simulink model "COHERENT_MODEM_WITH_LOGIC"  (R2021b)
settings: Solver=VariableStepAuto  StartTime=0.0  StopTime=0.04*5  RelTol=1e-3
values from neighbouring files (symbols this model uses):
  fcarrier = 20000    [run_modem.m]
libraries: dspswit3 x5, dsparch4 x2, simulink x1
settings Model: Creator=hp  LastModifiedBy=caccolillo
settings SolverCC: AlgebraicLoopSolver=TrustRegion
settings DataIOCC: ReturnWorkspaceOutputs=off
settings DebuggingCC: SFMachineParentedDataDiag=warning  ArithmeticOperatorsInVariantConditions=warning
settings SFSimCC: SimUseLocalCustomCode=off  CustomCodeUndefinedFunction=UseInterfaceOnly
settings RTWCC: RTWUseLocalCustomCode=off

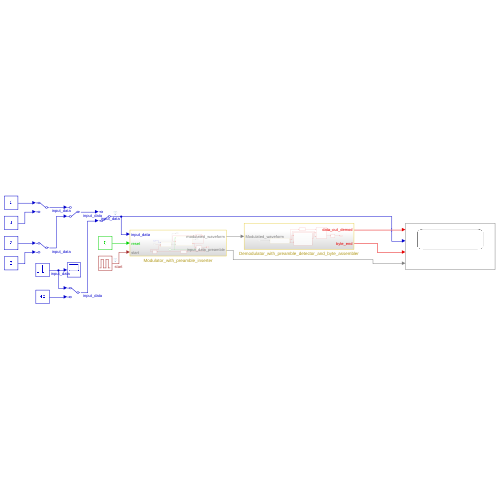
[thumbnail: Simulink's stored preview of the top-level diagram]
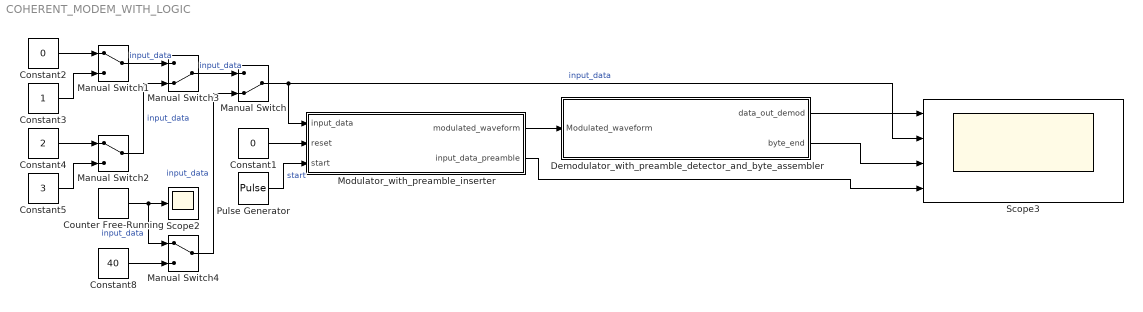
== system COHERENT_MODEM_WITH_LOGIC ==
  Constant1 : Constant  Value=0  OutDataTypeStr=double  SampleTime=1/20000
  Constant2 : Constant  Value=0  OutDataTypeStr=fixdt(0,2)  SampleTime=4/fcarrier
  Constant3 : Constant  OutDataTypeStr=fixdt(0,2)  SampleTime=4/fcarrier
  Constant4 : Constant  Value=2  OutDataTypeStr=fixdt(0,2)  SampleTime=4/fcarrier
  Constant5 : Constant  Value=3  OutDataTypeStr=fixdt(0,2)  SampleTime=4/fcarrier
  Constant8 : Constant  Value=40  OutDataTypeStr=fixdt(0,8)  SampleTime=4/fcarrier
  Counter Free-Running : simulink/Sources/Counter Free-Running  NumBits=8  tsamp=4/fcarrier
  Demodulator_with_preamble_detector_and_byte_assembler : Subsystem
  Manual Switch : ManualSwitch  CurrentSetting=0
  Manual Switch1 : ManualSwitch
  Manual Switch2 : ManualSwitch
  Manual Switch3 : ManualSwitch  CurrentSetting=0
  Manual Switch4 : ManualSwitch
  Modulator_with_preamble_inserter : Subsystem
  Pulse Generator : DiscretePulseGenerator  PulseType=Time based  Period=180/fcarrier  PulseWidth=5
  Scope2 : Scope
  Scope3 : Scope  NumInputPorts=4
  wires:
  Counter Free-Running/1 -> Scope2/1, Manual Switch4/1  "input_data"
  Pulse Generator/1 -> Modulator_with_preamble_inserter/3(start)  "start"
  Modulator_with_preamble_inserter/2(input_data_preamble) -> Scope3/4
  Demodulator_with_preamble_detector_and_byte_assembler/2(byte_end) -> Scope3/3
  Constant1/1 -> Modulator_with_preamble_inserter/2(reset)
  Modulator_with_preamble_inserter/1(modulated_waveform) -> Demodulator_with_preamble_detector_and_byte_assembler/1(Modulated_waveform)
  Manual Switch/1 -> Modulator_with_preamble_inserter/1(input_data), Scope3/2  "input_data"
  Manual Switch4/1 -> Manual Switch/2  "input_data"
  Constant4/1 -> Manual Switch2/1
  Demodulator_with_preamble_detector_and_byte_assembler/1(data_out_demod) -> Scope3/1
  Constant2/1 -> Manual Switch1/1
  Constant8/1 -> Manual Switch4/2
  Constant5/1 -> Manual Switch2/2
  Constant3/1 -> Manual Switch1/2
  Manual Switch3/1 -> Manual Switch/1  "input_data"
  Manual Switch2/1 -> Manual Switch3/2  "input_data"
  Manual Switch1/1 -> Manual Switch3/1  "input_data"

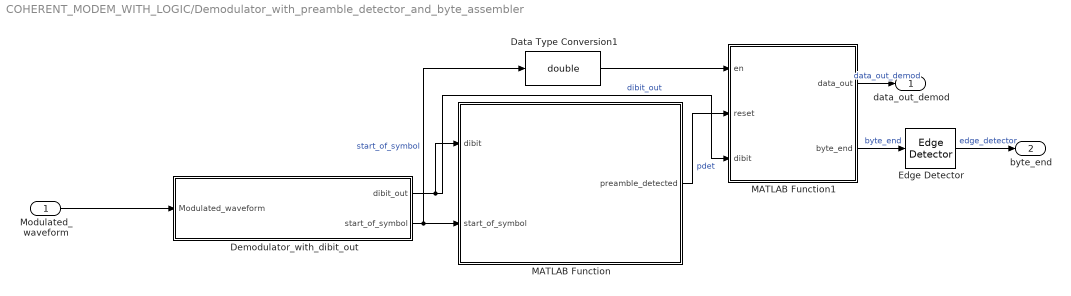
== system COHERENT_MODEM_WITH_LOGIC/Demodulator_with_preamble_detector_and_byte_assembler ==
  Modulated_waveform : Inport
  Data Type Conversion1 : DataTypeConversion  OutDataTypeStr=double
  Demodulator_with_dibit_out : Subsystem
  Edge Detector : dspswit3/Edge Detector  InputProcessing=Columns as channels (frame based)
      settings: SourceProductBaseCode=DS
  MATLAB Function : MATLAB Function  TreatAsAtomicUnit=on
  MATLAB Function1 : MATLAB Function  TreatAsAtomicUnit=on
  data_out_demod : Outport
  byte_end : Outport  Port=2
  wires:
  Demodulator_with_dibit_out/1(dibit_out) -> MATLAB Function/1(dibit), MATLAB Function1/3(dibit)  "dibit_out"
  Demodulator_with_dibit_out/2(start_of_symbol) -> MATLAB Function/2(start_of_symbol), Data Type Conversion1/1  "start_of_symbol"
  Edge Detector/1 -> byte_end/1  "edge_detector"
  Modulated_waveform/1 -> Demodulator_with_dibit_out/1(Modulated_waveform)
  MATLAB Function/1(preamble_detected) -> MATLAB Function1/2(reset)  "pdet"
  Data Type Conversion1/1 -> MATLAB Function1/1(en)
  MATLAB Function1/1(data_out) -> data_out_demod/1  "data_out_demod"
  MATLAB Function1/2(byte_end) -> Edge Detector/1  "byte_end"

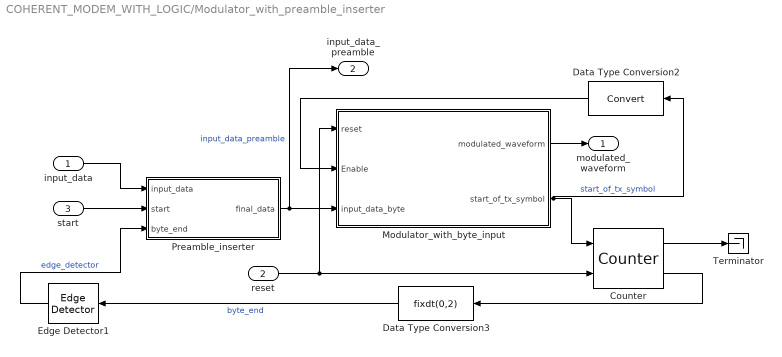
== system COHERENT_MODEM_WITH_LOGIC/Modulator_with_preamble_inserter ==
  input_data : Inport
  reset : Inport  Port=2
  start : Inport  Port=3
  Counter : dspswit3/Counter  Direction=Up  CountEvent=Rising edge  CounterSize=User defined  MaxCount=7  InitialCount=0  Output=Count and Hit  HitValue=7  ResetInput=on  SamplesPerFrame=1  Ts=1  CntDtype=double  HitDtype=Logical
  Data Type Conversion2 : DataTypeConversion
  Data Type Conversion3 : DataTypeConversion  OutMin=[0]  OutMax=[1]  OutDataTypeStr=fixdt(0,2)
  Edge Detector1 : dspswit3/Edge Detector  InputProcessing=Columns as channels (frame based)
      settings: SourceProductBaseCode=DS
  Modulator_with_byte_input : Subsystem
  Preamble_inserter : Subsystem
  Terminator : Terminator
  modulated_waveform : Outport
  input_data_preamble : Outport  Port=2
  wires:
  Preamble_inserter/1(final_data) -> Modulator_with_byte_input/3(input_data_byte), input_data_preamble/1  "input_data_preamble"
  reset/1 -> Counter/2, Modulator_with_byte_input/1(reset)
  Counter/2 -> Data Type Conversion3/1
  Counter/1 -> Terminator/1
  Edge Detector1/1 -> Preamble_inserter/3(byte_end)  "edge_detector"
  start/1 -> Preamble_inserter/2(start)
  Modulator_with_byte_input/2(start_of_tx_symbol) -> Counter/1, Data Type Conversion2/1  "start_of_tx_symbol"
  input_data/1 -> Preamble_inserter/1(input_data)
  Data Type Conversion3/1 -> Edge Detector1/1  "byte_end"
  Data Type Conversion2/1 -> Modulator_with_byte_input/2(Enable)
  Modulator_with_byte_input/1(modulated_waveform) -> modulated_waveform/1

== system COHERENT_MODEM_WITH_LOGIC/Demodulator_with_preamble_detector_and_byte_assembler/Demodulator_with_dibit_out ==
  Modulated_waveform : Inport
  Convert_to_decimal : Subsystem
  Demodulator_with_output_register : Subsystem
  dibit_out : Outport
  start_of_symbol : Outport  Port=2
  wires:
  Demodulator_with_output_register/1(i_demod) -> Convert_to_decimal/2(bit1)
  Demodulator_with_output_register/2(q_demod) -> Convert_to_decimal/1(bit0)
  Convert_to_decimal/1(convert) -> dibit_out/1  "dibit_out"
  Demodulator_with_output_register/3(start_of_symbol) -> start_of_symbol/1
  Modulated_waveform/1 -> Demodulator_with_output_register/1(Modulated_waveform)

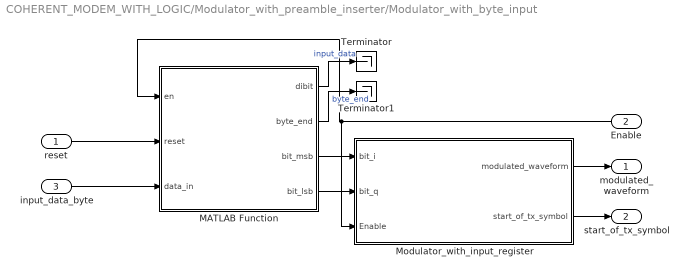
== system COHERENT_MODEM_WITH_LOGIC/Modulator_with_preamble_inserter/Modulator_with_byte_input ==
  reset : Inport
  Enable : Inport  Port=2
  input_data_byte : Inport  Port=3
  MATLAB Function : MATLAB Function  TreatAsAtomicUnit=on
  Modulator_with_input_register : Subsystem
  Terminator : Terminator
  Terminator1 : Terminator
  modulated_waveform : Outport
  start_of_tx_symbol : Outport  Port=2
  wires:
  Enable/1 -> MATLAB Function/1(en), Modulator_with_input_register/3(Enable)
  MATLAB Function/2(byte_end) -> Terminator1/1  "byte_end"
  Modulator_with_input_register/2(start_of_tx_symbol) -> start_of_tx_symbol/1
  input_data_byte/1 -> MATLAB Function/3(data_in)
  reset/1 -> MATLAB Function/2(reset)
  MATLAB Function/1(dibit) -> Terminator/1  "input_data"
  MATLAB Function/4(bit_lsb) -> Modulator_with_input_register/2(bit_q)
  Modulator_with_input_register/1(modulated_waveform) -> modulated_waveform/1
  MATLAB Function/3(bit_msb) -> Modulator_with_input_register/1(bit_i)

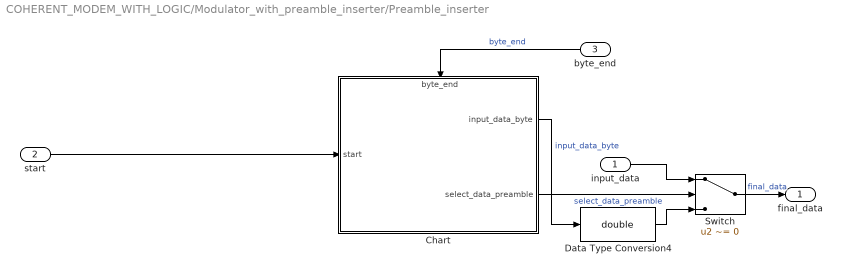
== system COHERENT_MODEM_WITH_LOGIC/Modulator_with_preamble_inserter/Preamble_inserter ==
  input_data : Inport
  start : Inport  Port=2
  byte_end : Inport  Port=3
  Chart : Stateflow chart  TreatAsAtomicUnit=on
      settings: PortSchema="{\"entries\":[{\"content\":{\"sides\":[{\"content\":{\"connectorIds\":[\"In2\"]},\"type\":\"ConnectorPlacement.EquallySpacedRectSide\",\"uuid\":\"c7ea0b9c-d106-4bd1-82e3-4c4e9722273c\"},{\"content\":{\"connectorIds\":[\"Out1\",\"Out2\"],\"side\":\"RIGHT\"},\"type\":\"ConnectorPlacement.EquallySpacedRectSide\",\"uuid\":\"4cc951b6-537b-4e23-ae77-107cf1cb9d20\"},{\"content\":{\"connectorIds\":[\"In1\"],\"side\":\"TOP\"},\"type\":\"ConnectorPlacement.EquallySpacedRectSide\",\"uuid\":\"96187a88-f84a-4d19-a7a7-49870645ca9d\"}]},\"type\":\"ConnectorPlacement.EquallySpacedConnector\",\"uuid\":\"a478a027-a6f7-4a96-ae1b-a22c0dc62afa\"}],\"packageUris\":[\"http://schema.mathworks.com/mf0/Connector/R2020b\"],\"version\":\"1.0\"}"
  Data Type Conversion4 : DataTypeConversion  OutMin=[0]  OutMax=[1]  OutDataTypeStr=double
  Switch : Switch  Criteria=u2 ~= 0  Threshold=1
  final_data : Outport
  wires:
  Switch/1 -> final_data/1  "final_data"
  input_data/1 -> Switch/1
  Data Type Conversion4/1 -> Switch/3
  Chart/2(select_data_preamble) -> Switch/2  "select_data_preamble"
  byte_end/1 -> Chart/1(byte_end)  "byte_end"
  Chart/1(input_data_byte) -> Data Type Conversion4/1  "input_data_byte"
  start/1 -> Chart/2(start)

== system COHERENT_MODEM_WITH_LOGIC/Demodulator_with_preamble_detector_and_byte_assembler/Demodulator_with_dibit_out/Convert_to_decimal ==
  bit0 : Inport
  bit1 : Inport  Port=2
  Add : Sum
  Gain1 : Gain  Gain=2
  convert : Outport
  wires:
  bit1/1 -> Gain1/1
  bit0/1 -> Add/1
  Add/1 -> convert/1  "convert"
  Gain1/1 -> Add/2

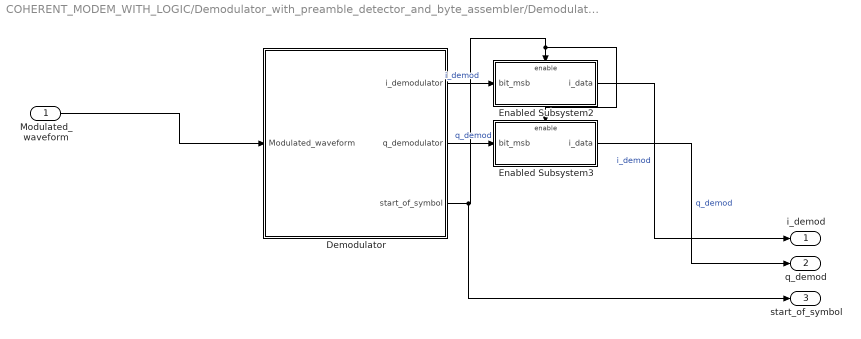
== system COHERENT_MODEM_WITH_LOGIC/Demodulator_with_preamble_detector_and_byte_assembler/Demodulator_with_dibit_out/Demodulator_with_output_register ==
  Modulated_waveform : Inport
  Demodulator : Subsystem
  Enabled Subsystem2 : Subsystem  TreatAsAtomicUnit=on
  Enabled Subsystem3 : Subsystem  TreatAsAtomicUnit=on
  i_demod : Outport
  q_demod : Outport  Port=2
  start_of_symbol : Outport  Port=3
  wires:
  Demodulator/2(q_demodulator) -> Enabled Subsystem3/1(bit_msb)  "q_demod"
  Demodulator/3(start_of_symbol) -> start_of_symbol/1, Enabled Subsystem3/Enable, Enabled Subsystem2/Enable
  Modulated_waveform/1 -> Demodulator/1(Modulated_waveform)
  Demodulator/1(i_demodulator) -> Enabled Subsystem2/1(bit_msb)  "i_demod"
  Enabled Subsystem2/1(i_data) -> i_demod/1  "i_demod"
  Enabled Subsystem3/1(i_data) -> q_demod/1  "q_demod"

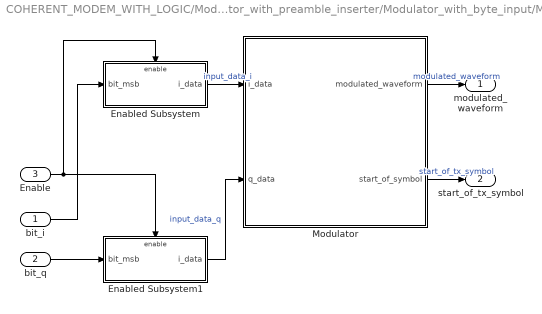
== system COHERENT_MODEM_WITH_LOGIC/Modulator_with_preamble_inserter/Modulator_with_byte_input/Modulator_with_input_register ==
  bit_i : Inport
  bit_q : Inport  Port=2
  Enable : Inport  Port=3
  Enabled Subsystem : Subsystem  TreatAsAtomicUnit=on
  Enabled Subsystem1 : Subsystem  TreatAsAtomicUnit=on
  Modulator : Subsystem
  modulated_waveform : Outport
  start_of_tx_symbol : Outport  Port=2
  wires:
  Enabled Subsystem/1(i_data) -> Modulator/1(i_data)  "input_data_i"
  Modulator/2(start_of_symbol) -> start_of_tx_symbol/1  "start_of_tx_symbol"
  bit_q/1 -> Enabled Subsystem1/1(bit_msb)
  bit_i/1 -> Enabled Subsystem/1(bit_msb)
  Enabled Subsystem1/1(i_data) -> Modulator/2(q_data)  "input_data_q"
  Modulator/1(modulated_waveform) -> modulated_waveform/1  "modulated_waveform"
  Enable/1 -> Enabled Subsystem/Enable, Enabled Subsystem1/Enable

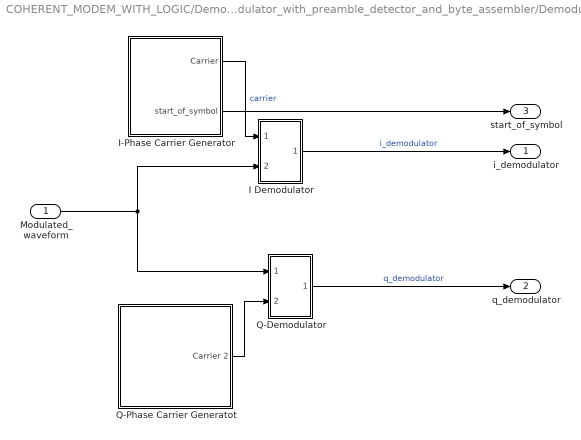
== system COHERENT_MODEM_WITH_LOGIC/Demodulator_with_preamble_detector_and_byte_assembler/Demodulator_with_dibit_out/Demodulator_with_output_register/Demodulator ==
  Modulated_waveform : Inport
  "I Demodulator " : Subsystem
  "I-Phase Carrier Generator " : Subsystem
  Q-Demodulator : Subsystem
  Q-Phase Carrier Generatot : Subsystem
  i_demodulator : Outport
  q_demodulator : Outport  Port=2
  start_of_symbol : Outport  Port=3
  wires:
  Q-Demodulator/1(Out1) -> q_demodulator/1  "q_demodulator"
  Modulated_waveform/1 -> Q-Demodulator/1(In1), "I Demodulator "/2(In2)
  Q-Phase Carrier Generatot/1("Carrier 2 ") -> Q-Demodulator/2("Carrier 2 ")
  "I Demodulator "/1(Out1) -> i_demodulator/1  "i_demodulator"
  "I-Phase Carrier Generator "/1(Carrier) -> "I Demodulator "/1(Carrier)  "carrier"
  "I-Phase Carrier Generator "/2(start_of_symbol) -> start_of_symbol/1

== system COHERENT_MODEM_WITH_LOGIC/Demodulator_with_preamble_detector_and_byte_assembler/Demodulator_with_dibit_out/Demodulator_with_output_register/Enabled Subsystem2 ==
  bit_msb : Inport
  Enable : EnablePort
  i_data : Outport
  wires:
  bit_msb/1 -> i_data/1

== system COHERENT_MODEM_WITH_LOGIC/Demodulator_with_preamble_detector_and_byte_assembler/Demodulator_with_dibit_out/Demodulator_with_output_register/Enabled Subsystem3 ==
  bit_msb : Inport
  Enable : EnablePort
  i_data : Outport
  wires:
  bit_msb/1 -> i_data/1

== system COHERENT_MODEM_WITH_LOGIC/Modulator_with_preamble_inserter/Modulator_with_byte_input/Modulator_with_input_register/Enabled Subsystem ==
  bit_msb : Inport
  Enable : EnablePort
  i_data : Outport
  wires:
  bit_msb/1 -> i_data/1

== system COHERENT_MODEM_WITH_LOGIC/Modulator_with_preamble_inserter/Modulator_with_byte_input/Modulator_with_input_register/Enabled Subsystem1 ==
  bit_msb : Inport
  Enable : EnablePort
  i_data : Outport
  wires:
  bit_msb/1 -> i_data/1

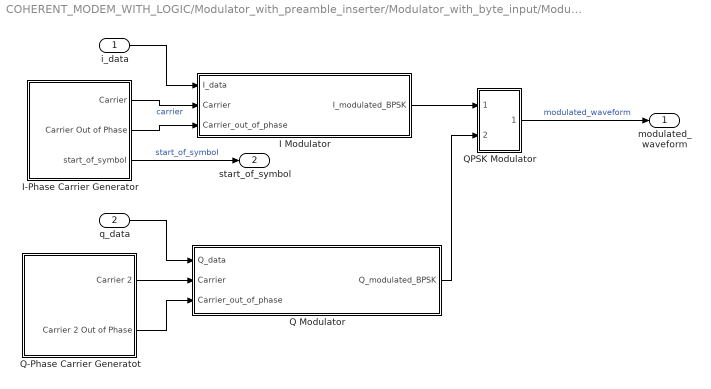
== system COHERENT_MODEM_WITH_LOGIC/Modulator_with_preamble_inserter/Modulator_with_byte_input/Modulator_with_input_register/Modulator ==
  i_data : Inport
  q_data : Inport  Port=2
  I Modulator : Subsystem
  "I-Phase Carrier Generator " : Subsystem
  Q Modulator : Subsystem
  Q-Phase Carrier Generatot : Subsystem
  QPSK Modulator : Subsystem
  modulated_waveform : Outport
  start_of_symbol : Outport  Port=2
  wires:
  I Modulator/1(I_modulated_BPSK) -> QPSK Modulator/1(In1)
  q_data/1 -> Q Modulator/1(Q_data)
  i_data/1 -> I Modulator/1(I_data)
  Q Modulator/1("Q_modulated_BPSK ") -> QPSK Modulator/2(In2)
  QPSK Modulator/1(Out1) -> modulated_waveform/1  "modulated_waveform"
  "I-Phase Carrier Generator "/2("Carrier Out of Phase ") -> I Modulator/3(Carrier_out_of_phase)
  Q-Phase Carrier Generatot/1("Carrier 2 ") -> Q Modulator/2(Carrier)
  Q-Phase Carrier Generatot/2(Carrier 2 Out of Phase) -> Q Modulator/3(Carrier_out_of_phase)
  "I-Phase Carrier Generator "/1(Carrier) -> I Modulator/2(Carrier)  "carrier"
  "I-Phase Carrier Generator "/3(start_of_symbol) -> start_of_symbol/1  "start_of_symbol"

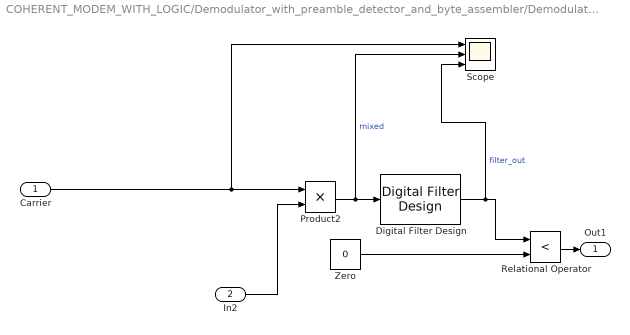
== system COHERENT_MODEM_WITH_LOGIC/Demodulator_with_preamble_detector_and_byte_assembler/Demodulator_with_dibit_out/Demodulator_with_output_register/Demodulator/I Demodulator  ==
  Carrier : Inport
  In2 : Inport  Port=2
  Digital Filter Design : dsparch4/Digital Filter Design  mwdsp_browser_bugfix_var=off
  Product2 : Product
  Relational Operator : RelationalOperator  Operator=<  OutDataTypeStr=boolean  RndMeth=Simplest
  Scope : Scope  NumInputPorts=3
  Zero : Constant  Value=0
  Out1 : Outport  VectorParamsAs1DForOutWhenUnconnected=off
  wires:
  Digital Filter Design/1 -> Scope/3, Relational Operator/1  "filter_out"
  In2/1 -> Product2/2
  Product2/1 -> Scope/2, Digital Filter Design/1  "mixed"
  Zero/1 -> Relational Operator/2
  Relational Operator/1 -> Out1/1
  Carrier/1 -> Scope/1, Product2/1

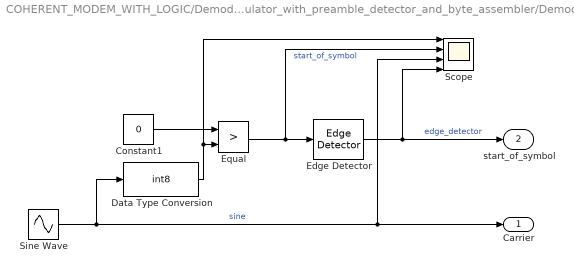
== system COHERENT_MODEM_WITH_LOGIC/Demodulator_with_preamble_detector_and_byte_assembler/Demodulator_with_dibit_out/Demodulator_with_output_register/Demodulator/I-Phase Carrier Generator  ==
  Constant1 : Constant  Value=0  OutDataTypeStr=int8
  Data Type Conversion : DataTypeConversion  OutDataTypeStr=int8
  Edge Detector : dspswit3/Edge Detector  InputProcessing=Columns as channels (frame based)
      settings: SourceProductBaseCode=DS
  Equal : RelationalOperator  Operator=>  OutDataTypeStr=boolean  RndMeth=Simplest
  Scope : Scope  NumInputPorts=4
  Sine Wave : Sin  Frequency=2*pi*fcarrier  SampleTime=1/(100*fcarrier)
  Carrier : Outport  VectorParamsAs1DForOutWhenUnconnected=off
  start_of_symbol : Outport  Port=2
  wires:
  Constant1/1 -> Equal/1
  Equal/1 -> Scope/2, Edge Detector/1  "start_of_symbol"
  Data Type Conversion/1 -> Scope/1, Equal/2
  Edge Detector/1 -> Scope/4, start_of_symbol/1  "edge_detector"
  Sine Wave/1 -> Data Type Conversion/1, Scope/3, Carrier/1  "sine"

== system COHERENT_MODEM_WITH_LOGIC/Demodulator_with_preamble_detector_and_byte_assembler/Demodulator_with_dibit_out/Demodulator_with_output_register/Demodulator/Q-Demodulator ==
  In1 : Inport
  "Carrier 2 " : Inport  Port=2
  Digital Filter Design1 : dsparch4/Digital Filter Design  mwdsp_browser_bugfix_var=off
  Product3 : Product
  Relational Operator1 : RelationalOperator  Operator=<  OutDataTypeStr=boolean  RndMeth=Simplest
  Zero1 : Constant  Value=0
  Out1 : Outport  VectorParamsAs1DForOutWhenUnconnected=off
  wires:
  Zero1/1 -> Relational Operator1/2
  Digital Filter Design1/1 -> Relational Operator1/1
  Product3/1 -> Digital Filter Design1/1
  "Carrier 2 "/1 -> Product3/1
  Relational Operator1/1 -> Out1/1
  In1/1 -> Product3/2

== system COHERENT_MODEM_WITH_LOGIC/Demodulator_with_preamble_detector_and_byte_assembler/Demodulator_with_dibit_out/Demodulator_with_output_register/Demodulator/Q-Phase Carrier Generatot ==
  Sine Wave1 : Sin  Frequency=2*pi*fcarrier  Phase=pi/2  SampleTime=1/(100*fcarrier)
  "Carrier 2 " : Outport  VectorParamsAs1DForOutWhenUnconnected=off
  wires:
  Sine Wave1/1 -> "Carrier 2 "/1

== system COHERENT_MODEM_WITH_LOGIC/Modulator_with_preamble_inserter/Modulator_with_byte_input/Modulator_with_input_register/Modulator/I Modulator ==
  I_data : Inport
  Carrier : Inport  Port=2
  Carrier_out_of_phase : Inport  Port=3
  Switch : Switch  Criteria=u2 > Threshold  Threshold=0.5
  I_modulated_BPSK : Outport  VectorParamsAs1DForOutWhenUnconnected=off
  wires:
  Carrier/1 -> Switch/3
  Carrier_out_of_phase/1 -> Switch/1
  I_data/1 -> Switch/2
  Switch/1 -> I_modulated_BPSK/1

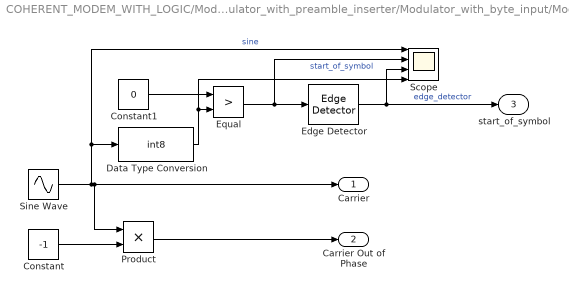
== system COHERENT_MODEM_WITH_LOGIC/Modulator_with_preamble_inserter/Modulator_with_byte_input/Modulator_with_input_register/Modulator/I-Phase Carrier Generator  ==
  Constant : Constant  Value=-1
  Constant1 : Constant  Value=0  OutDataTypeStr=int8
  Data Type Conversion : DataTypeConversion  OutDataTypeStr=int8  SaturateOnIntegerOverflow=on
  Edge Detector : dspswit3/Edge Detector  InputProcessing=Columns as channels (frame based)
      settings: SourceProductBaseCode=DS
  Equal : RelationalOperator  Operator=>  OutDataTypeStr=boolean  RndMeth=Simplest
  Product : Product
  Scope : Scope  NumInputPorts=4
  Sine Wave : Sin  Frequency=2*pi*fcarrier  SampleTime=1/(100*fcarrier)
  Carrier : Outport  VectorParamsAs1DForOutWhenUnconnected=off
  "Carrier Out of Phase " : Outport  Port=2  VectorParamsAs1DForOutWhenUnconnected=off
  start_of_symbol : Outport  Port=3
  wires:
  Constant/1 -> Product/2
  Product/1 -> "Carrier Out of Phase "/1
  Sine Wave/1 -> Carrier/1, Product/1, Scope/1, Data Type Conversion/1  "sine"
  Equal/1 -> Scope/2, Edge Detector/1  "start_of_symbol"
  Constant1/1 -> Equal/1
  Data Type Conversion/1 -> Scope/4, Equal/2
  Edge Detector/1 -> Scope/3, start_of_symbol/1  "edge_detector"

== system COHERENT_MODEM_WITH_LOGIC/Modulator_with_preamble_inserter/Modulator_with_byte_input/Modulator_with_input_register/Modulator/Q Modulator ==
  Q_data : Inport
  Carrier : Inport  Port=2
  Carrier_out_of_phase : Inport  Port=3
  Switch1 : Switch  Criteria=u2 > Threshold  Threshold=0.5
  "Q_modulated_BPSK " : Outport  VectorParamsAs1DForOutWhenUnconnected=off
  wires:
  Q_data/1 -> Switch1/2
  Carrier_out_of_phase/1 -> Switch1/1
  Switch1/1 -> "Q_modulated_BPSK "/1
  Carrier/1 -> Switch1/3

== system COHERENT_MODEM_WITH_LOGIC/Modulator_with_preamble_inserter/Modulator_with_byte_input/Modulator_with_input_register/Modulator/Q-Phase Carrier Generatot ==
  Constant1 : Constant  Value=-1
  Product1 : Product
  Sine Wave1 : Sin  Frequency=2*pi*fcarrier  Phase=pi/2  SampleTime=1/(100*fcarrier)
  "Carrier 2 " : Outport  VectorParamsAs1DForOutWhenUnconnected=off
  Carrier 2 Out of Phase : Outport  Port=2  VectorParamsAs1DForOutWhenUnconnected=off
  wires:
  Constant1/1 -> Product1/2
  Sine Wave1/1 -> Product1/1, "Carrier 2 "/1
  Product1/1 -> Carrier 2 Out of Phase/1

== system COHERENT_MODEM_WITH_LOGIC/Modulator_with_preamble_inserter/Modulator_with_byte_input/Modulator_with_input_register/Modulator/QPSK Modulator ==
  In1 : Inport
  In2 : Inport  Port=2
  Add : Sum
  Out1 : Outport  VectorParamsAs1DForOutWhenUnconnected=off
  wires:
  In2/1 -> Add/2
  In1/1 -> Add/1
  Add/1 -> Out1/1

== matlab function COHERENT_MODEM_WITH_LOGIC/Demodulator_with_preamble_detector_and_byte_assembler/MATLAB Function ==
  data: dibit input; preamble_detected output; start_of_symbol input
function preamble_detected = detect_preamble(dibit, start_of_symbol)
%DETECT_PREAMBLE Detects a run of at least 31 consecutive dibit==2,
%followed by dibit==3 (only evaluated when start_of_symbol == 1).
%
% State Machine:
%   State 0: Counting consecutive dibit==2
%            → If count >= 31, transition to State 1
%   State 1: Stay in this state as long as dibit==2
%            → If dibit==3, trigger detection and reset
%            → Else, reset

    % Persistent state and counter
    persistent state count_two
    if isempty(state)
        state = 0;
        count_two = 0;
    end

    % Default output
    preamble_detected = false;

    if start_of_symbol == 1
        switch state
            case 0
                if dibit == 2
                    count_two = count_two + 1;
                    if count_two >= 31
                        state = 1; % Start monitoring for dibit==3
                    end
                else
                    count_two = 0;
                end

            case 1
                if dibit == 2
                    % Stay in this state, continue accepting more 2s
                    % No change to count_two
                elseif dibit == 3
                    % Preamble matched
                    preamble_detected = true;
                    % Reset
                    state = 0;
                    count_two = 0;
                else
                    % Invalid sequence; reset
                    state = 0;
                    count_two = 0;
                end
        end
    end
end

== stateflow chart COHERENT_MODEM_WITH_LOGIC/Modulator_with_preamble_inserter/Preamble_inserter/Chart ==
  state wait_start
    input_data_byte=0;
    select_data_preamble=1;
  state wait_byte_end
    input_data_byte=0;
    select_data_preamble=1;
  state send_start_of_data1
    input_data_byte=170;
    select_data_preamble=0;
  state send_stop_of_data2
    input_data_byte=170;
    select_data_preamble=0;
  state send_stop_of_data3
    input_data_byte=170;
    select_data_preamble=0;
  state send_start_of_data4
    input_data_byte=170;
    select_data_preamble=0;
  state send_start_of_data5
    input_data_byte=170;
    select_data_preamble=0;
  state send_stop_of_frame_delimiter1
    input_data_byte=171;
    select_data_preamble=0;
  note: [byte_end== 1 ]
  state send_stop_of_data7
    input_data_byte=170;
    select_data_preamble=0;
  state send_stop_of_data6
    input_data_byte=170;
    select_data_preamble=0;
  (default) -> wait_start
  wait_start -> wait_byte_end : [start==1]
  wait_byte_end -> send_start_of_data1 : [byte_end==1]
  send_stop_of_frame_delimiter1 -> wait_start : [byte_end==1]
  send_stop_of_data3 -> send_start_of_data4 : [byte_end==1]
  send_start_of_data1 -> send_stop_of_data2 : [byte_end==1]
  send_start_of_data4 -> send_start_of_data5 : [byte_end==1]
  send_stop_of_data2 -> send_stop_of_data3 : [byte_end==1]
  send_start_of_data5 -> send_stop_of_data6 : [byte_end==1]
  send_stop_of_data7 -> send_stop_of_frame_delimiter1
  send_stop_of_data6 -> send_stop_of_data7 : [byte_end==1]
  data: byte_end input; start input; input_data_byte output; select_data_preamble output

== matlab function COHERENT_MODEM_WITH_LOGIC/Modulator_with_preamble_inserter/Modulator_with_byte_input/MATLAB Function ==
  data: en input; dibit output; reset input; data_in input; byte_end output; bit_msb output; bit_lsb output
function [dibit, byte_end, bit_msb, bit_lsb] = dibit_extractor(en, reset, data_in)
% dibit_extractor  Extracts two-bit segments from an 8-bit input on enable pulses
%   en        : boolean enable signal (rising edge triggers output update)
%   reset     : boolean reset signal (synchronous reset of internal state)
%   data_in   : uint8 8-bit input data
%   dibit     : UFix_2_0 2-bit unsigned fixed-point output
%   byte_end  : real scalar; goes high every four dibits (i.e., end of byte)
%   bit_msb   : logical scalar; the most-significant bit of the dibit
%   bit_lsb   : logical scalar; the least-significant bit of the dibit

%#codegen

persistent count prev_en
if isempty(count)
    count   = uint8(3);   % cycle index (0 to 3)
    prev_en = 0;          % previous enable state
end

% Default outputs
byte_end = 0;
bit_msb  = false;
bit_lsb  = false;

% Synchronous reset
if reset
    count = uint8(0);
else
    % Detect rising edge of enable
    if en == 1 && prev_en == 0
        % Increment and wrap count
        count = mod(count + 1, 4);

        % Pulse byte_end when completing the fourth dibit
        if count == 1
            byte_end = 1;
        end
    end
end

prev_en = en;

% Determine starting bit position (0-based)
startBit = count * 2;

% Extract two bits (MATLAB bitget uses 1-based positions)
bit0 = bitget(data_in, startBit + 1);  % LSB of the dibit
bit1 = bitget(data_in, startBit + 2);  % MSB of the dibit

% Expose individual bits as Booleans
bit_lsb = logical(bit0);
bit_msb = logical(bit1);

% Assemble value (bit1 is MSB, bit0 is LSB)
value = uint8(bit1) * 2 + uint8(bit0);

% Create 2-bit unsigned fixed-point output
dibit = fi(value, 0, 2, 0);
end

== matlab function COHERENT_MODEM_WITH_LOGIC/Demodulator_with_preamble_detector_and_byte_assembler/MATLAB Function1 ==
  data: en input; data_out output; reset input; dibit input; byte_end output
function [data_out,byte_end] = byte_assembler(en, reset, dibit)
% byte_assembler  Assembles 8-bit data from four 2-bit segments
%   en        : boolean enable signal (rising edge triggers input sampling)
%   reset     : boolean reset signal (synchronous reset of internal state)
%   dibit     : ufix2 2-bit input
%   data_out  : uint8 8-bit output, valid after 4 dibits

%#codegen

persistent count temp_byte prev_en
if isempty(count)
    count = uint8(0);
    temp_byte = uint8(0);
    prev_en = 0;
    byte_end = 0;
end

% Synchronous reset
if reset
    count = uint8(1);
    temp_byte = uint8(0);
    byte_end = 0;
end

% Detect rising edge of enable
if en==1 && prev_en==0 && reset==0
    shift = bitshift(uint8(dibit), count * 2);  % Place dibit at the correct position
    mask = bitshift(uint8(3), count * 2);       % Create mask for clearing that position
    temp_byte = bitor(bitand(temp_byte, bitcmp(mask, 'uint8')), shift);

    % Increment count and wrap
    count = mod(count + 1, 4);
end
prev_en = en;

% Output the assembled byte only when 4 dibits have been collected
if count == 0 && reset==0
    data_out = temp_byte;
    byte_end = 1;
else
    data_out = uint8(0);
    byte_end = 0;
end
end
